simulink library "Lib_Turbo_PGenerator_TMATS_org"  (Simulink 10.0)
settings: Solver=ode45  StartTime=0.0  StopTime=10.0  RelTol=1e-3  EnableMultiTasking=on
Description:
  | Thomas Modules
settings Model: Creator=jwchapm2  LastModifiedBy=bhisma

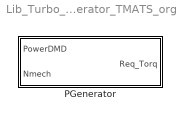
== system Lib_Turbo_PGenerator_TMATS_org ==
  PGenerator : Subsystem  mask(T-MATS: Power Generation Library Block){Eff_M=.995}
      mask prompts: Eff_M "Eff_M - Efficiency"
      mask help: This block converts a power demand with rotational speed into a torque and can be used to simulate a power generator.
      mask Help: web(which('Turbo_TMATS_PGen.html'),'-helpbrowser')

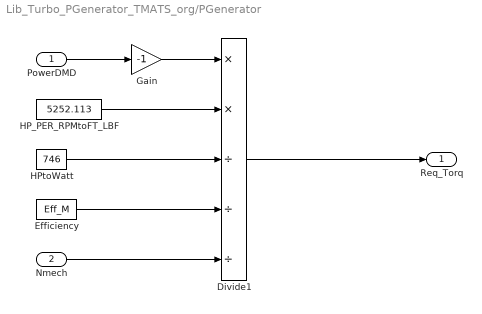
== system Lib_Turbo_PGenerator_TMATS_org/PGenerator ==
  PowerDMD : Inport
  Nmech : Inport  Port=2
  Divide1 : Product  Inputs=**///
  Efficiency : Constant  Value=Eff_M
  Gain : Gain  Gain=-1
  HP_PER_RPMtoFT_LBF : Constant  Value=5252.113
  HPtoWatt : Constant  Value=746
  Req_Torq : Outport
  wires:
  PowerDMD/1 -> Gain/1
  Divide1/1 -> Req_Torq/1
  Nmech/1 -> Divide1/5
  Gain/1 -> Divide1/1
  HPtoWatt/1 -> Divide1/3
  HP_PER_RPMtoFT_LBF/1 -> Divide1/2
  Efficiency/1 -> Divide1/4
